simulink model "equacoesMIC2"  (R2023a)
settings: Solver=VariableStepAuto  StartTime=0.0  StopTime=16  RelTol=1e-3
libraries: simulink x1
settings Model: Creator=Aluno - LPR 3  LastModifiedBy=Aluno - LPR 6

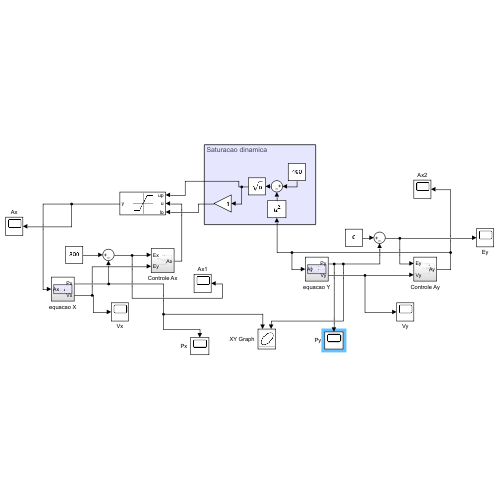
[thumbnail: Simulink's stored preview of the top-level diagram]
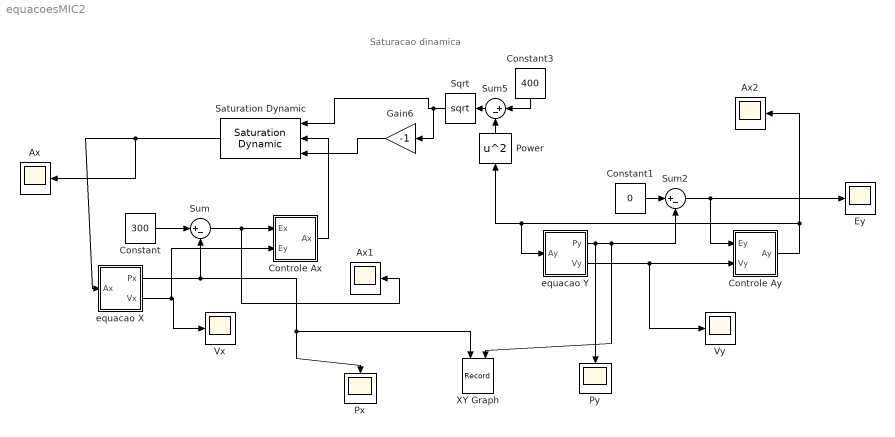
== system equacoesMIC2 ==
  note: Saturacao dinamica
  Ax : Scope
  Ax1 : Scope
  Ax2 : Scope
  Constant : Constant  Value=300
  Constant1 : Constant  Value=0
  Constant3 : Constant  Value=400
  Controle Ax : Subsystem
  Controle Ay : Subsystem
  Ey : Scope
  Gain6 : Gain  Gain=-1
  Power : Math  Operator=square
  Px : Scope
  Py : Scope
  Saturation Dynamic : simulink/Discontinuities/Saturation Dynamic  OutMin=[]  OutMax=[]  OutDataTypeStr=Inherit: Same as second input  OutDataType=fixdt(1, 16)  OutScaling=2^-10  DoSatur=off
  Sqrt : Sqrt
  Sum : Sum  Inputs=|+-
  Sum2 : Sum  Inputs=|+-
  Sum5 : Sum  Inputs=|+-
  Vx : Scope
  Vy : Scope
  XY Graph : Record  FileSettingsInternal="{\"entries\":[{\"content\":{\"excelSettings\":{\"content\":{},\"type\":\"Streamout.ExcelSettings\"}},\"type\":\"Streamout.FileSettingStorage\",\"uuid\":\"1f06f097-43c7-4b81-bbc7-2c9f697b8832\"}],\"packageUris\":[\"http://schema.mathworks.com/mf0/streamout_blocks/R2020a\"],\"version\":\"1.0\"}"  Layout=[1 1]  SignalsInternal="{\"entries\":[{\"content\":{\"signals\":[{\"content\":{\"blockPath\":[\"equacoesMIC2/XY Graph\"],\"dimensions\":[1],\"domain\":\"equacoesMIC2/XY Graph\",\"lineColor\":\"#a2142f\",\"plots\":[1],\"port\":1,\"sid\":[\"\"],\"signalID\":217002,\"signalName\":\"equacao X:1\"},\"type\":\"RecordBlkView.Signal\",\"uuid\":\"5a1bc97a-f328-4992-ab4d-956ca500140f\"},{\"content\":{\"blockPath\":[\"equacoesMIC2/XY Graph\"],\"dimensions\":[1],\"domain\":\"equacoesMIC2/XY Graph\",\"lineColor\":\"#139fff\",\"plots\":[1],\"port\":2,\"sid\":[\"\"],\"signalID\":217006,\"signalName\":\"equacao Y:1\"},\"type\":\"RecordBlkView.Signal\",\"uuid\":\"fc31a20c-af5d-4821-b790-ed8e7926dc79\"}]},\"type\":\"RecordBlkView.InputSignals\",\"uuid\":\"f3717547-be67-4a3d-9eb9-6f2dc5f70525\"}],\"packageUris\":[\"http://schema.mathworks.com/mf0/streamout_blocks/R2020a\"],\"version\":\"1.0\"}"  VisualizationBindings="{\"xyplotplugin\":{\"info\":[{\"series\":[{\"bindingParametersList\":[{\"parameter\":\"X-Axis\",\"signalID\":217002,\"signalName\":\"equacao X:1\"},{\"parameter\":\"Y-Axis\",\"signalID\":217006,\"signalName\":\"equacao Y:1\"}],\"seriesID\":35863}],\"subplotID\":1}]}}"  CompatibilityTag=XY
  equacao X : Subsystem
  equacao Y : Subsystem
  wires:
  Constant/1 -> Sum/1
  equacao X/1(Px) -> XY Graph/1, Px/1, Sum/2
  Saturation Dynamic/1 -> Ax/1, equacao X/1(Ax)
  equacao Y/1(Py) -> XY Graph/2, Sum2/2, Py/1
  Constant1/1 -> Sum2/1
  Sum2/1 -> Ey/1, Controle Ay/1(Ey)
  Sqrt/1 -> Saturation Dynamic/1, Gain6/1
  Gain6/1 -> Saturation Dynamic/3
  Sum/1 -> Ax1/1, Controle Ax/1(Ex)
  equacao X/2(Vx) -> Vx/1, Controle Ax/2(Ey)
  Controle Ax/1(Ax) -> Saturation Dynamic/2
  equacao Y/2(Vy) -> Vy/1, Controle Ay/2(Vy)
  Constant3/1 -> Sum5/1
  Sum5/1 -> Sqrt/1
  Power/1 -> Sum5/2
  Controle Ay/1(Ay) -> Power/1, equacao Y/1(Ay), Ax2/1

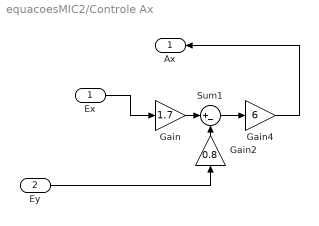
== system equacoesMIC2/Controle Ax ==
  Ex : Inport
  Ey : Inport  Port=2
  Gain : Gain  Gain=1.7
  Gain2 : Gain  Gain=0.8
  Gain4 : Gain  Gain=6
  Sum1 : Sum  Inputs=|+-
  Ax : Outport
  wires:
  Gain2/1 -> Sum1/2
  Sum1/1 -> Gain4/1
  Gain/1 -> Sum1/1
  Ex/1 -> Gain/1
  Gain4/1 -> Ax/1
  Ey/1 -> Gain2/1

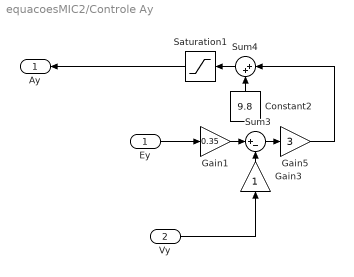
== system equacoesMIC2/Controle Ay ==
  Ey : Inport
  Vy : Inport  Port=2
  Constant2 : Constant  Value=9.8
  Gain1 : Gain  Gain=0.35
  Gain3 : Gain
  Gain5 : Gain  Gain=3
  Saturation1 : Saturate  UpperLimit=11  LowerLimit=-11
  Sum3 : Sum  Inputs=|+-
  Sum4 : Sum  Inputs=|++
  Ay : Outport
  wires:
  Gain3/1 -> Sum3/2
  Ey/1 -> Gain1/1
  Sum3/1 -> Gain5/1
  Gain5/1 -> Sum4/1
  Gain1/1 -> Sum3/1
  Sum4/1 -> Saturation1/1
  Constant2/1 -> Sum4/2
  Saturation1/1 -> Ay/1
  Vy/1 -> Gain3/1

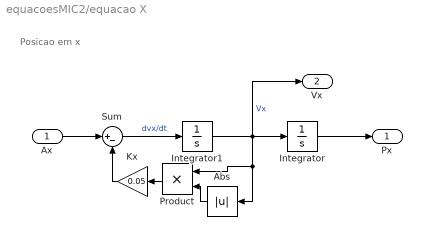
== system equacoesMIC2/equacao X ==
  note: Posicao em x
  Ax : Inport
  Abs : Abs  SaturateOnIntegerOverflow=off
  Integrator : Integrator  InitialCondition=45
  Integrator1 : Integrator  InitialCondition=13.2
  Kx : Gain  Gain=0.05
  Product : Product
  Sum : Sum  Inputs=|+-
  Px : Outport
  Vx : Outport  Port=2
  wires:
  Integrator1/1 -> Product/1, Abs/1, Vx/1, Integrator/1  "Vx"
  Ax/1 -> Sum/1
  Integrator/1 -> Px/1
  Kx/1 -> Sum/2
  Sum/1 -> Integrator1/1  "dvx/dt"
  Product/1 -> Kx/1
  Abs/1 -> Product/2

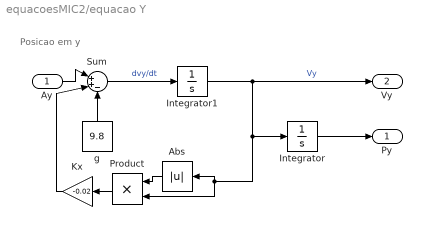
== system equacoesMIC2/equacao Y ==
  note: Posicao em y
  Ay : Inport
  Abs : Abs  SaturateOnIntegerOverflow=off
  Integrator : Integrator  InitialCondition=40
  Integrator1 : Integrator  InitialCondition=-14.74
  Kx : Gain  Gain=-0.02
  Product : Product
  Sum : Sum  Inputs=|++-
  g : Constant  Value=9.8
  Py : Outport
  Vy : Outport  Port=2
  wires:
  Integrator1/1 -> Vy/1, Product/2, Abs/1, Integrator/1  "Vy"
  Ay/1 -> Sum/1
  Kx/1 -> Sum/2
  g/1 -> Sum/3
  Sum/1 -> Integrator1/1  "dvy/dt"
  Integrator/1 -> Py/1
  Product/1 -> Kx/1
  Abs/1 -> Product/1
